simulink model "week2problem4"  (R2020b)
settings: Solver=VariableStepAuto  StartTime=0.0  StopTime=10.0  RelTol=1e-3
model workspace (MAT data in the model file):
  Ke = 0
  Kt = 0
  L = 2.75
  R = 4
  Var4 = 0
undefined symbols (not defined in the file): Kd, Ki, Kp
settings Model: Creator=HP  LastModifiedBy=HP

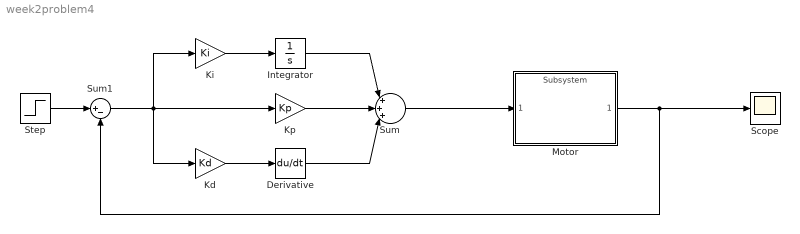
== system week2problem4 ==
  Derivative : Derivative
  Integrator : Integrator
  Kd : Gain  Gain=Kd
  Ki : Gain  Gain=Ki
  Kp : Gain  Gain=Kp
  Motor : ModelReference  ModelNameDialog=Subsystem  SimulationMode=Normal  ModelReferenceVersion=1.7
  Scope : Scope
  Step : Step  SampleTime=0
  Sum : Sum  Inputs=|+++|
  Sum1 : Sum  Inputs=|+-
  wires:
  Step/1 -> Sum1/1
  Integrator/1 -> Sum/1
  Kd/1 -> Derivative/1
  Ki/1 -> Integrator/1
  Sum/1 -> Motor/1
  Kp/1 -> Sum/2
  Motor/1 -> Sum1/2, Scope/1
  Sum1/1 -> Ki/1, Kd/1, Kp/1
  Derivative/1 -> Sum/3
